simulink library "apparentWind_ul"  (R2018b)
settings: Solver=VariableStepAuto  StartTime=0.0  StopTime=10.0  RelTol=1e-3
settings Model: Creator=mcobb  LastModifiedBy=mcobb

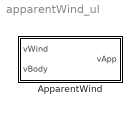
== system apparentWind_ul ==
  ApparentWind : Subsystem

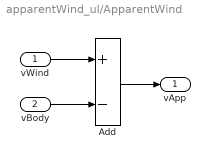
== system apparentWind_ul/ApparentWind ==
  vWind : Inport
  vBody : Inport  Port=2
  Add : Sum  Inputs=+-
  vApp : Outport
  wires:
  vBody/1 -> Add/2
  vWind/1 -> Add/1
  Add/1 -> vApp/1
